simulink model "Model_simulink_dyskretny"  (R2015a)
settings: Solver=ode3  SolverMode=SingleTasking  StartTime=0.0  StopTime=20  FixedStep=Tp  RelTol=1e-3
undefined symbols (not defined in the file): In, J, K2, Kp, Kt, Kw, Lambda, Mn, psi, Rt, T, Tp, Un, Uz0, wn, Y
settings Model: Creator=user  LastModifiedBy=user
settings DataIOCC: SignalLoggingSaveFormat=ModelDataLogs
settings OptimizationCC: BlockReduction=off  BooleanDataType=off  ExpressionDepthLimit=2147483647
settings DebuggingCC: SaveWithParameterizedLinksMsg=none  UnderspecifiedInitializationDetection=Classic  MergeDetectMultiDrivingBlocksExec=none  SignalResolutionControl=TryResolveAllWithWarning  MultiTaskDSMMsg=warning  MultiTaskCondExecSysMsg=none  StateNameClashWarn=warning
settings HardwareCC: TargetUnknown=on

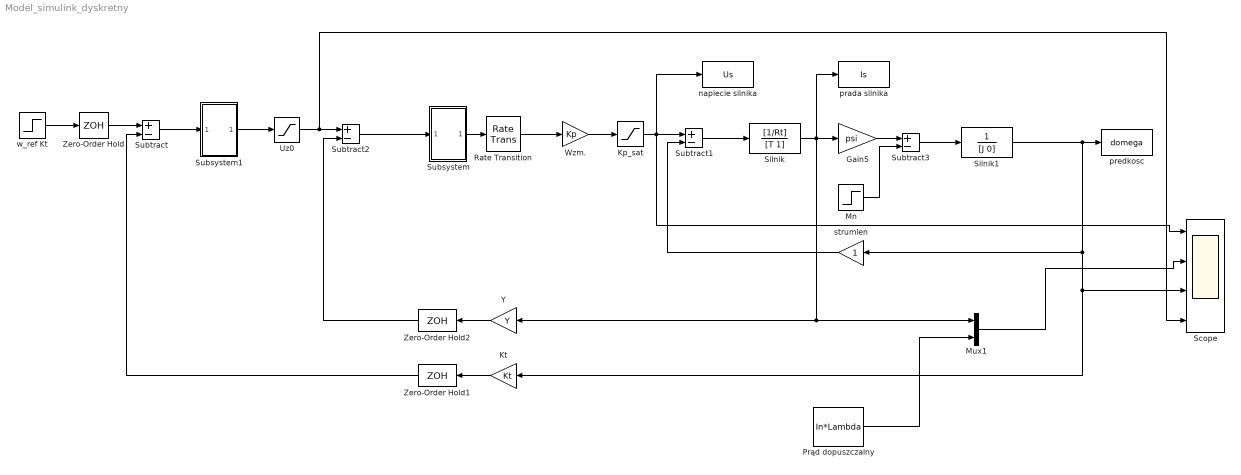
== system Model_simulink_dyskretny ==
  Gain5 : Gain  Gain=psi
  Kp_sat : Saturate  UpperLimit=1.5*Un  LowerLimit=-1.5*Un
  Kt : Gain  Gain=Kt
  Mn : Step  After=Mn  SampleTime=0
  Mux1 : Mux  Inputs=2
  Prąd dopuszczalny : Constant  Value=In*Lambda
  Rate Transition : RateTransition
  Scope : Scope  NumInputPorts=4
      settings: YMin=-5~-5~-5~-5  YMax=5~5~5~5
  Silnik : TransferFcn  Numerator=[1/Rt]  Denominator=[T 1]
  Silnik1 : TransferFcn  Numerator=1  Denominator=[J 0]
  Subsystem : Subsystem
  Subsystem1 : Subsystem
  Subtract{,1..3} (4 alike) : Sum  Inputs=+-
  Uz0 : Saturate  UpperLimit=Uz0  LowerLimit=-Uz0
  Wzm. : Gain  Gain=Kp
  Y : Gain  Gain=Y
  Zero-Order Hold : ZeroOrderHold
  Zero-Order Hold1 : ZeroOrderHold  SampleTime=Tp
  Zero-Order Hold2 : ZeroOrderHold  SampleTime=Tp
  napiecie silnika : ToWorkspace  VariableName=Us  SaveFormat=Timeseries  SampleTime=-1
  prada silnika : ToWorkspace  VariableName=Is  SaveFormat=Timeseries  SampleTime=-1
  predkosc : ToWorkspace  VariableName=domega  SaveFormat=Timeseries  SampleTime=-1
  strumien : Gain
  w_ref Kt : Step  Before=wn*Kt  After=wn*Kt  SampleTime=0
  wires:
  Wzm./1 -> Kp_sat/1
  Subtract1/1 -> Silnik/1
  Silnik/1 -> prada silnika/1, Y/1, Mux1/1, Gain5/1
  Gain5/1 -> Subtract3/1
  Subtract3/1 -> Silnik1/1
  Mn/1 -> Subtract3/2
  strumien/1 -> Subtract1/2
  Kp_sat/1 -> Scope/1, napiecie silnika/1, Subtract1/1
  Mux1/1 -> Scope/2
  Prąd dopuszczalny/1 -> Mux1/2
  Uz0/1 -> Scope/4, Subtract2/1
  Silnik1/1 -> predkosc/1, strumien/1, Kt/1, Scope/3
  w_ref Kt/1 -> Zero-Order Hold/1
  Zero-Order Hold/1 -> Subtract/1
  Kt/1 -> Zero-Order Hold1/1
  Zero-Order Hold1/1 -> Subtract/2
  Subtract2/1 -> Subsystem/1(In1)
  Subsystem1/1(Out1) -> Uz0/1
  Subtract/1 -> Subsystem1/1(In1)
  Subsystem/1(Out1) -> Rate Transition/1
  Rate Transition/1 -> Wzm./1
  Y/1 -> Zero-Order Hold2/1
  Zero-Order Hold2/1 -> Subtract2/2

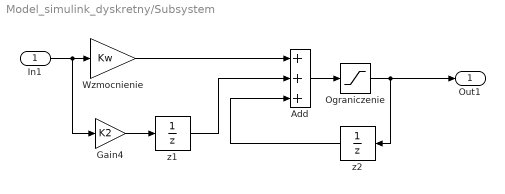
== system Model_simulink_dyskretny/Subsystem ==
  In1 : Inport
  Add : Sum  Inputs=+++
  Gain4 : Gain  Gain=K2
  Ograniczenie : Saturate
  Wzmocnienie : Gain  Gain=Kw
  z1 : UnitDelay  SampleTime=-1
  z2 : UnitDelay  SampleTime=-1
  Out1 : Outport
  wires:
  In1/1 -> Gain4/1, Wzmocnienie/1
  Wzmocnienie/1 -> Add/1
  Gain4/1 -> z1/1
  z1/1 -> Add/2
  Add/1 -> Ograniczenie/1
  Ograniczenie/1 -> Out1/1, z2/1
  z2/1 -> Add/3

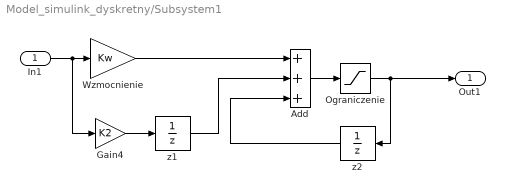
== system Model_simulink_dyskretny/Subsystem1 ==
  In1 : Inport
  Add : Sum  Inputs=+++
  Gain4 : Gain  Gain=K2
  Ograniczenie : Saturate
  Wzmocnienie : Gain  Gain=Kw
  z1 : UnitDelay  SampleTime=Tp
  z2 : UnitDelay  SampleTime=Tp
  Out1 : Outport
  wires:
  In1/1 -> Gain4/1, Wzmocnienie/1
  Wzmocnienie/1 -> Add/1
  Gain4/1 -> z1/1
  z1/1 -> Add/2
  Add/1 -> Ograniczenie/1
  Ograniczenie/1 -> Out1/1, z2/1
  z2/1 -> Add/3
